simulink model "system_1st_order_ff"  (R2018b)
settings: Solver=ode8  StartTime=0.0  StopTime=5  FixedStep=0.01  RelTol=1e-3
settings Model: Creator=suvo.ganguli  LastModifiedBy=GW00174198

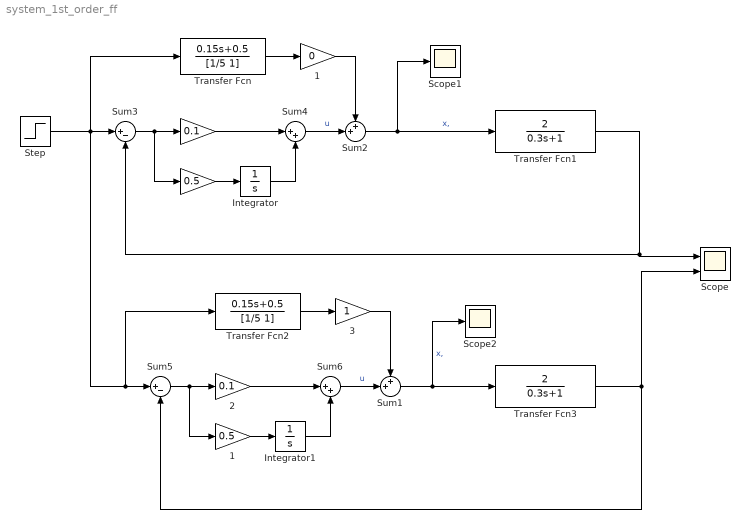
== system system_1st_order_ff ==
  " " : Gain  Gain=0.5
  "  " : Gain  Gain=0.1
  "  1" : Gain  Gain=0
  "  2" : Gain  Gain=0.1
  "  3" : Gain
  " 1" : Gain  Gain=0.5
  Integrator : Integrator
  Integrator1 : Integrator
  Scope : Scope  NumInputPorts=2
  Scope1 : Scope
  Scope2 : Scope
  Step : Step  SampleTime=0
  Sum1 : Sum  Inputs=++|
  Sum2 : Sum  Inputs=++|
  Sum3 : Sum  Inputs=|+-
  Sum4 : Sum  Inputs=|++
  Sum5 : Sum  Inputs=|+-
  Sum6 : Sum  Inputs=|++
  Transfer Fcn : TransferFcn  Numerator=[0.15 0.5]  Denominator=[1/5 1]
  Transfer Fcn1 : TransferFcn  Numerator=[2]  Denominator=[0.3 1]
  Transfer Fcn2 : TransferFcn  Numerator=[0.15 0.5]  Denominator=[1/5 1]
  Transfer Fcn3 : TransferFcn  Numerator=[2]  Denominator=[0.3 1]
  wires:
  Sum2/1 -> Transfer Fcn1/1, Scope1/1  "x,"
  Transfer Fcn1/1 -> Sum3/2, Scope/1
  Transfer Fcn/1 -> "  1"/1
  " "/1 -> Integrator/1
  Integrator/1 -> Sum4/2
  "  "/1 -> Sum4/1
  Sum3/1 -> " "/1, "  "/1
  Sum4/1 -> Sum2/2  "u"
  "  1"/1 -> Sum2/1
  "  3"/1 -> Sum1/1
  Step/1 -> Sum5/1, Transfer Fcn2/1, Transfer Fcn/1, Sum3/1
  Sum6/1 -> Sum1/2  "u"
  Sum5/1 -> "  2"/1, " 1"/1
  "  2"/1 -> Sum6/1
  Integrator1/1 -> Sum6/2
  " 1"/1 -> Integrator1/1
  Transfer Fcn2/1 -> "  3"/1
  Transfer Fcn3/1 -> Scope/2, Sum5/2
  Sum1/1 -> Scope2/1, Transfer Fcn3/1  "x,"
